simulink model "ovi"  (R2015b)
settings: Solver=VariableStepAuto  StartTime=0.0  StopTime=2.0  RelTol=1e-3
settings Model: Creator=ovi  LastModifiedBy=ovi

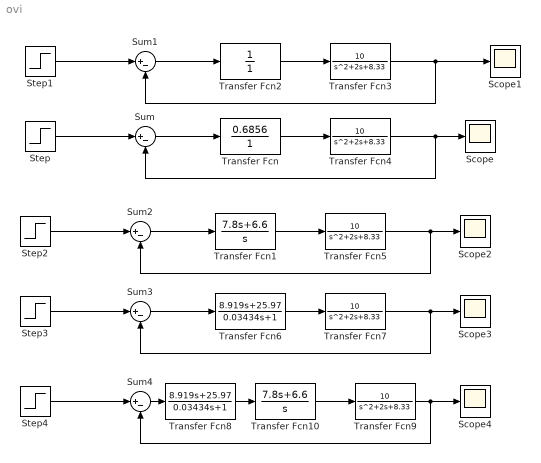
== system ovi ==
  Scope{,1..4} (5 alike) : Scope
  Step{,1..3} (4 alike) : Step  SampleTime=0
  Step4 : Step  Time=0.5  SampleTime=0
  Sum{,1..4} (5 alike) : Sum  Inputs=|+-
  Transfer Fcn : TransferFcn  Numerator=[0.6856]  Denominator=[1]
  Transfer Fcn1 : TransferFcn  Numerator=[7.8 6.6]  Denominator=[1 0]
  Transfer Fcn10 : TransferFcn  Numerator=[7.8 6.6]  Denominator=[1 0]
  Transfer Fcn2 : TransferFcn  Denominator=[1]
  Transfer Fcn{3..5,7,9} (5 alike) : TransferFcn  Numerator=[10]  Denominator=[1 2 8.33]
  Transfer Fcn6 : TransferFcn  Numerator=[8.919 25.97]  Denominator=[0.03434 1]
  Transfer Fcn8 : TransferFcn  Numerator=[8.919 25.97]  Denominator=[0.03434 1]
  wires:
  Transfer Fcn/1 -> Transfer Fcn4/1
  Step/1 -> Sum/1
  Sum/1 -> Transfer Fcn/1
  Transfer Fcn4/1 -> Sum/2, Scope/1
  Transfer Fcn2/1 -> Transfer Fcn3/1
  Step1/1 -> Sum1/1
  Sum1/1 -> Transfer Fcn2/1
  Transfer Fcn3/1 -> Sum1/2, Scope1/1
  Transfer Fcn1/1 -> Transfer Fcn5/1
  Step2/1 -> Sum2/1
  Sum2/1 -> Transfer Fcn1/1
  Transfer Fcn5/1 -> Sum2/2, Scope2/1
  Transfer Fcn6/1 -> Transfer Fcn7/1
  Step3/1 -> Sum3/1
  Sum3/1 -> Transfer Fcn6/1
  Transfer Fcn7/1 -> Sum3/2, Scope3/1
  Transfer Fcn8/1 -> Transfer Fcn10/1
  Step4/1 -> Sum4/1
  Sum4/1 -> Transfer Fcn8/1
  Transfer Fcn9/1 -> Sum4/2, Scope4/1
  Transfer Fcn10/1 -> Transfer Fcn9/1
